simulink model "untitled"  (R2014b)
settings: Solver=ode45  StartTime=0.0  StopTime=10.0  RelTol=1e-3
settings Model: Creator=PC  LastModifiedBy=Asus

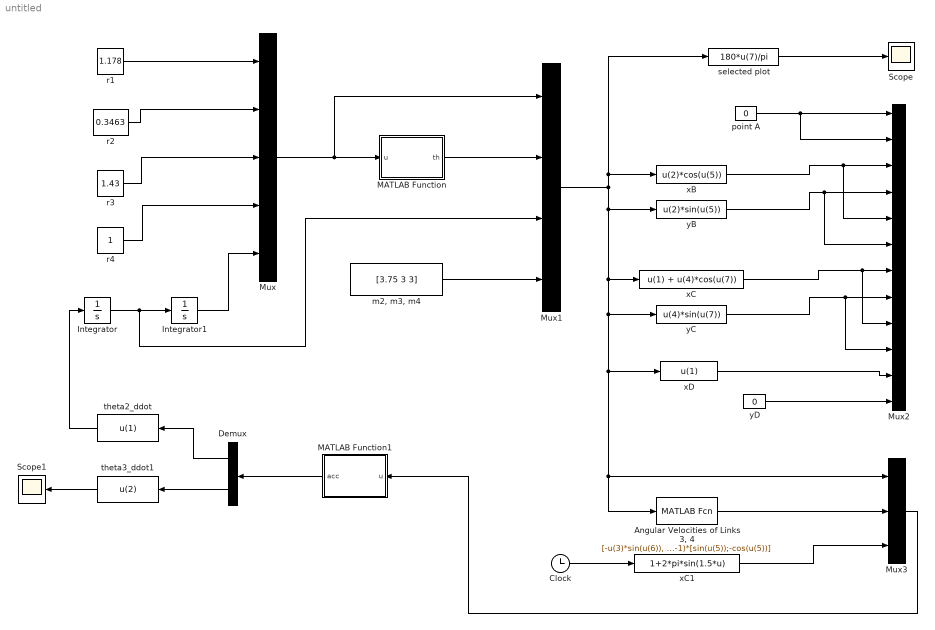
== system untitled ==
  "Angular Velocities of Links 3, 4" : MATLABFcn  MATLABFcn=[-u(3)*sin(u(6)), u(4)*sin(u(7)); u(3)*cos(u(6)), -u(4)*cos(u(7))]^(-1)*[sin(u(5));-cos(u(5))]  OutputDimensions=2
  Clock : Clock
  Demux : Demux  Outputs=2
  Integrator : Integrator
  Integrator1 : Integrator
  MATLAB Function : MATLAB Function  TreatAsAtomicUnit=on
  MATLAB Function1 : MATLAB Function  TreatAsAtomicUnit=on
  Mux : Mux  Inputs=5
  Mux1 : Mux
  Mux2 : Mux  Inputs=12
  Mux3 : Mux  Inputs=3
  Scope : Scope
  Scope1 : Scope
  "m2, m3, m4" : Constant  Value=[3.75 3 3]
  point A : Constant  Value=0
  r1 : Constant  Value=1.178
  r2 : Constant  Value=0.3463
  r3 : Constant  Value=1.43
  r4 : Constant
  selected plot : Fcn  Expr=180*u(7)/pi
  theta2_ddot : Fcn  Expr=u(1)
  theta3_ddot1 : Fcn  Expr=u(2)
  xB : Fcn  Expr=u(2)*cos(u(5))
  xC : Fcn  Expr=u(1) + u(4)*cos(u(7))
  xC1 : Fcn  Expr=1+2*pi*sin(1.5*u)
  xD : Fcn  Expr=u(1)
  yB : Fcn  Expr=u(2)*sin(u(5))
  yC : Fcn  Expr=u(4)*sin(u(7))
  yD : Constant  Value=0
  wires:
  r1/1 -> Mux/1
  r2/1 -> Mux/2
  r3/1 -> Mux/3
  r4/1 -> Mux/4
  Mux/1 -> Mux1/1, MATLAB Function/1(u)
  MATLAB Function/1(th) -> Mux1/2
  Integrator1/1 -> Mux/5
  Integrator/1 -> Mux1/3, Integrator1/1
  "m2, m3, m4"/1 -> Mux1/4
  MATLAB Function1/1(acc) -> Demux/1
  point A/1 -> Mux2/2, Mux2/1
  xB/1 -> Mux2/5, Mux2/3
  yB/1 -> Mux2/6, Mux2/4
  xC/1 -> Mux2/9, Mux2/7
  yC/1 -> Mux2/10, Mux2/8
  xD/1 -> Mux2/11
  yD/1 -> Mux2/12
  selected plot/1 -> Scope/1
  Mux1/1 -> "Angular Velocities of Links 3, 4"/1, Mux3/1, xD/1, yC/1, xC/1, yB/1, selected plot/1, xB/1
  xC1/1 -> Mux3/3
  Clock/1 -> xC1/1
  Mux3/1 -> MATLAB Function1/1(u)
  Demux/2 -> theta3_ddot1/1
  Demux/1 -> theta2_ddot/1
  theta3_ddot1/1 -> Scope1/1
  theta2_ddot/1 -> Integrator/1
  "Angular Velocities of Links 3, 4"/1 -> Mux3/2

== matlab function untitled/MATLAB Function1 ==
  data: u input; acc output
function acc  = accel(u)
A =[1/3*u(9)*u(2)^2 0 0 u(2)*sin(u(5)) -u(2)*cos(u(5));
    0 1/3*u(10)*u(3)^2 -1/2*u(10)*u(3)*u(4)*cos(u(7)-u(6)) u(3)*sin(u(6)) - u(3)*cos(u(6));
    0 -1/2*u(10)*u(3)*u(4)*cos(u(7)-u(6)) (1/3*u(11)+u(10))*u(4)^2 - u(4)*sin(u(7)) u(4)*cos(u(7));
    u(2)*sin(u(5)) u(3)*sin(u(6)) -u(4)*sin(u(7)) 0 0; 
    u(2)*cos(u(5)) u(3)*cos(u(6)) -u(4)*cos(u(7)) 0 0]
B = [u(14); 
    -1/2*u(10)*u(3)*u(4)*u(13)^2*sin(u(7)-u(6));
    1/2*u(10)*u(3)*u(4)*u(12)^2*sin(u(7)-u(6));
    u(4)*u(13)^2*cos(u(7))-u(3)*u(12)^2*cos(u(6))-u(2)*u(8)^2*cos(u(5));
    -u(4)*u(13)^2*sin(u(7))+u(3)*u(12)^2*sin(u(6))+u(2)*u(8)^2*sin(u(5))]
acc = (A^-1)*B
end

== matlab function untitled/MATLAB Function ==
  data: u input; th output
function th =Newton(u)
factor=pi/180;
theta2=u(5);
theta3=45*factor;
theta4=135*factor;
f=[u(3)*cos(theta3)-u(4)*cos(theta4)+u(2)*cos(theta2)-u(1);
u(3)*sin(theta3)-u(4)*sin(theta4)+u(2)*sin(theta2)];
while norm(f)>1.0E-6
    Jacobian=[-u(3)*sin(theta3) u(4)*sin(theta4); u(3)*cos(theta3) - u(4)*cos(theta4)];
    delta= inv(Jacobian)*-1*f;
    theta3=theta3+delta(1);
    theta4=theta4+delta(2);
    f=[u(3)*cos(theta3)-u(4)*cos(theta4)+u(2)*cos(theta2)-u(1);
    u(3)*sin(theta3)-u(4)*sin(theta4)+u(2)*sin(theta2)];
    norm(f);
end;
th(1)=theta3;
th(2)=theta4;
